simulink model "secondmodel"  (R2018b)
settings: Solver=VariableStepAuto  StartTime=0.0  StopTime=10.0  RelTol=1e-3
values from neighbouring files (symbols this model uses):
  x = input(" Enter your choice: ")    [systemtest.m]
settings Model: Creator=Egypt_Laptop  LastModifiedBy=Egypt_Laptop

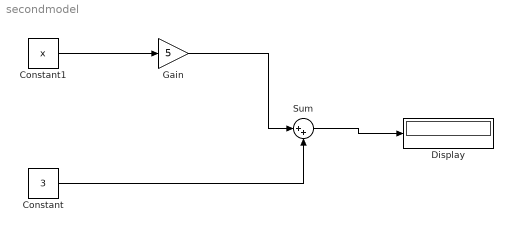
== system secondmodel ==
  Constant : Constant  Value=3
  Constant1 : Constant  Value=x
  Display : Display
  Gain : Gain  Gain=5
  Sum : Sum  Inputs=|++
  wires:
  Constant1/1 -> Gain/1
  Gain/1 -> Sum/1
  Constant/1 -> Sum/2
  Sum/1 -> Display/1
